simulink model "CB_sfun"  (R2024b)
settings: Solver=FixedStepDiscrete  StartTime=0.0  StopTime=inf  RelTol=1e-3  EnableMultiTasking=on
values from neighbouring files (symbols this model uses):
  cblc_battChargingMode = 5    [CB_ini.m]
  cblc_deltaSocThreshBalance = 0.1    [CB_ini.m]
  cblc_socThreshBalance = 50    [CB_ini.m]
settings Model: TunableVars=cblc_battChargingMode,cblc_deltaSocThreshBalance,cblc_socThreshBalance,cblc_voltThreshBalance  TunableVarsStorageClass=Auto,Auto,Auto,Auto  TunableVarsTypeQualifier=,,,  Creator=nctzv8  LastModifiedBy=voillat
settings ConfigSet: Description=OpenECU configuration set for code generation under RTW-EC.
settings SolverCC: AlgebraicLoopSolver=TrustRegion  PositivePriorityOrder=on
settings DataIOCC: LimitDataPoints=on  SaveFormat=Array  SignalLoggingSaveFormat=ModelDataLogs
settings OptimizationCC: DefaultParameterBehavior=Inlined  InlineInvariantSignals=on  ExpressionDepthLimit=2147483647  StateBitsets=on  DataBitsets=on  ZeroExternalMemoryAtStartup=off  ZeroInternalMemoryAtStartup=off  NoFixptDivByZeroProtection=on  EfficientFloat2IntCast=on  LifeSpan=1  EfficientTunableParamExpr=on
settings DebuggingCC: SaveWithParameterizedLinksMsg=none  SignalResolutionControl=TryResolveAllWithWarning  MultiTaskDSMMsg=warning  MultiTaskCondExecSysMsg=none  SingleTaskRateTransMsg=error  CheckMatrixSingularityMsg=warning  VectorMatrixConversionMsg=warning  SignalLabelMismatchMsg=warning  UnconnectedInputMsg=warning  UnconnectedOutputMsg=warning  UnconnectedLineMsg=warning  AllowSymbolicDim=off  StateNameClashWarn=warning  SFUnexpectedBacktrackingDiag=warning  SFNoUnconditionalDefaultTransitionDiag=warning  SFExecutionAtInitializationDiag=none  ArithmeticOperatorsInVariantConditions=warning
settings HardwareCC: ProdBitPerPointer=32  ProdBitPerSizeT=32  ProdBitPerPtrDiffT=32  ProdLargestAtomicInteger=Long  ProdLargestAtomicFloat=Double  ProdEndianess=BigEndian  ProdWordSize=32  ProdHWDeviceType=Freescale->32-bit PowerPC  TargetIntDivRoundTo=Zero  TargetEndianess=BigEndian  TargetHWDeviceType=Freescale->32-bit PowerPC  ProdEqTarget=off
settings ModelReferenceCC: EnableRefExpFcnMdlSchedulingChecks=on  PropagateSignalLabelsOutOfModel=off
settings SFSimCC: SimUseLocalCustomCode=off  MATLABDynamicMemAlloc=off  CustomCodeUndefinedFunction=UseInterfaceOnly
settings RTWCC: Description=OpenECU Platform Target (ERT, optimised floating-point code)  SystemTargetFile=openecu_ert.tlc  MakeCommand=make_rtw optimized_floating_point=1  TemplateMakefile=openecu_ert_r2015b_64.tmf  RetainRTWFile=on  RTWUseLocalCustomCode=off  IncludeHyperlinkInReport=on  GPUComputeCapability=3.5
settings CodeAppCC: ForceParamTrailComments=on  IgnoreCustomStorageClasses=off  SimulinkDataObjDesc=on  CustomSymbolStrType=$N$R$M  InsertBlockDesc=on  StateflowObjectComments=on  InternalIdentifier=Classic
settings STFCustomTargetCC: TargetLibSuffix=.a  GenerateSampleERTMain=on  IncludeMdlTerminateFcn=off  CombineOutputUpdateFcns=on  IncludeFileDelimiter=UseQuote  ERTCustomFileBanners=on  SupportContinuousTime=off  RemoveResetFunc=on  MATLABClassNameForMDSCustomization=Simulink.SoftwareTarget.ERTCustomization  SystemTargetFile=openecu_ert.tlc
settings ERTTargetCC: MultiwordLength=2048  GenerateSampleERTMain=on  ParMdlRefBuildCompliant=off  CompOptLevelCompliant=off  ConcurrentExecutionCompliant=off  IncludeMdlTerminateFcn=off  IncludeFileDelimiter=UseQuote  SupportNonInlinedSFcns=on  ModelStepFunctionPrototypeControlCompliant=off  CPPClassGenCompliant=off  UseToolchainInfoCompliant=off  ExtModeMexFile=noextcomm  ERTSrcFileBannerTemplate=oe_code_c_template.cgt  ERTHdrFileBannerTemplate=oe_code_h_template.cgt  ERTDataSrcFileTemplate=oe_data_c_template.cgt  ERTDataHdrFileTemplate=oe_data_h_template.cgt  ERTCustomFileTemplate=example_file_process.tlc  GlobalDataDefinition=InSeparateSourceFile  GlobalDataReference=InSeparateHeaderFile  ConvertIfToSwitch=off  SuppressUnreachableDefaultCases=off  EnableUserReplacementTypes=on  DynamicArrayContainerType=coder::array
settings ConfigComp: CovMetricSettings=dw  CovSaveCumulativeToWorkspaceVar=on  CovSaveSingleToWorkspaceVar=on  CovExternalEMLEnable=off

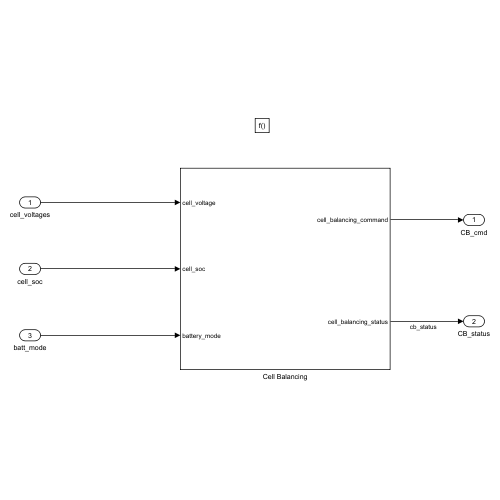
[thumbnail: Simulink's stored preview of the top-level diagram]
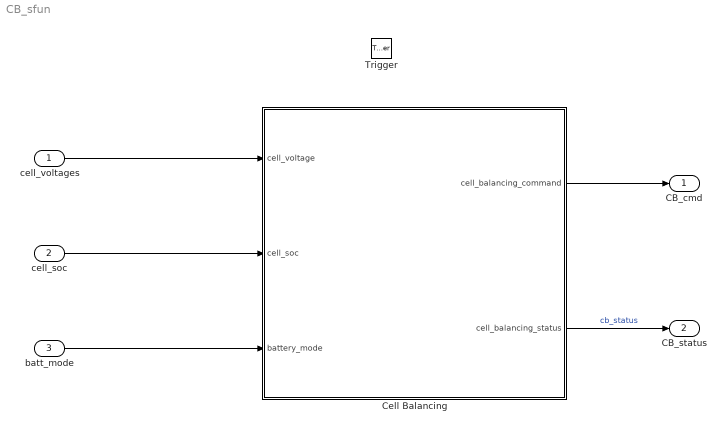
== system CB_sfun ==
  cell_voltages : Inport
  cell_soc : Inport  Port=2
  batt_mode : Inport  Port=3  OutDataTypeStr=uint8
  Trigger : TriggerPort  TriggerType=function-call  VariantControl=(inherit)  PortDimensions=1
  Cell Balancing : Subsystem  mask{sfcnParam1=cblc_battChargingMode, sfcnParam2=cblc_deltaSocThreshBalance, sfcnParam3=cblc_socThreshBalance}
      mask prompts: sfcnParam1 "cblc_battChargingMode:"; sfcnParam2 "cblc_deltaSocThreshBalance:"; sfcnParam3 "cblc_socThreshBalance:"
      mask help: Simulink:masks:GenSFuncDesc_MD
      mask Help: eval('feval(''rtwprivate'',''rtwhelpview'',''rtw_sfcn_block'')');
  CB_cmd : Outport
  CB_status : Outport  Port=2
  wires:
  cell_voltages/1 -> Cell Balancing/1(cell_voltage)
  batt_mode/1 -> Cell Balancing/3(battery_mode)
  cell_soc/1 -> Cell Balancing/2(cell_soc)
  Cell Balancing/1(cell_balancing_command) -> CB_cmd/1
  Cell Balancing/2(cell_balancing_status) -> CB_status/1  "cb_status"

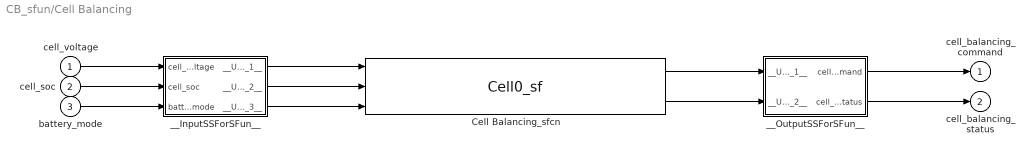
== system CB_sfun/Cell Balancing ==
  cell_voltage : Inport  PortDimensions=40
  cell_soc : Inport  Port=2  PortDimensions=40
  battery_mode : Inport  Port=3
  Cell Balancing_sfcn : S-Function  FunctionName=Cell0_sf  Parameters=sfcnParam1, sfcnParam2, sfcnParam3  SFunctionModules=""  SFunctionDeploymentMode=off  EnableBusSupport=off  mask{rtw_sf_name=Cell0_sf, showVar=off, sfcnParam1=sfcnParam1, sfcnParam2=sfcnParam2, sfcnParam3=sfcnParam3}
      mask prompts: rtw_sf_name "Simulink:masks:GenSFuncName_MP"; showVar "Simulink:masks:GenSFuncShowModuleList_MP"; sfcnParam1 "cblc_battChargingMode:"; sfcnParam2 "cblc_deltaSocThreshBalance:"; sfcnParam3 "cblc_socThreshBalance:"
      mask help: Simulink:masks:GenSFuncDesc_MD
      mask init:
      | displist = '';
      | if ~strcmp(get_param(gcb, 'FunctionName'), rtw_sf_name);
      |   set_param(gcb, 'FunctionName', rtw_sf_name);
      | end
      | % Check if we are generating code
      | rtw_mode = false;
      | if strcmpi(get_param(bdroot(gcb),'SimulationStatus'),'Initializing')
      | 	rtw_mode = strcmpi(get_param(bdroot(gcb),'BuildingRTWCode'),'on') && ...
      | 		~strcmpi(get_param(bdroot(gcb),'TargetStyle'),'SimulationTarget');
      | end
      | if showVar || rtw_mode
      | 	if exist('rtwsfunc') == 2 | exist('rtwsfunc') == 6
      | 		tmplist = rtwsfunc(rtw_sf_name,gcb);
      | 		tmplist = DAStudio.message('Simulink:masks:GenSFuncListOfModules_IC', tmplist);
      | 	elseif showVar
      | 		tmplist1 = DAStudio.message('Simulink:masks:GenSFuncListOfModules_IC', '');
      |         tmplist2 = DAStudio.message('Simulink:masks:GenSFuncNotLicensed_IC');
      |         tmplist = [tmplist1 tmplist2];
      |  	end
      | end
      | if showVar
      |   displist = tmplist;
      | end
      settings: CopyFcn=|
      | if ~strcmp(get_param(gcb,'Linkstatus'),'none') && ...
      | ~strcmp(get_param(gcb,'Linkstatus'),'implicit')
      |   set_param(gcb,'LinkStatus','none');
      | end
      mask Help: eval('feval(''rtwprivate'',''rtwhelpview'',''rtw_sfcn_block'')');
      mask Display:
      | port_label('input',1,'cell_voltage');
      | port_label('input',2,'cell_soc');
      | port_label('input',3,'battery_mode');
      | port_label('output',1,'cell_balancing_command');
      | port_label('output',2,'cell_balancing_status');
  __InputSSForSFun__ : Subsystem
  __OutputSSForSFun__ : Subsystem
  cell_balancing_command : Outport
  cell_balancing_status : Outport  Port=2
  wires:
  cell_voltage/1 -> __InputSSForSFun__/1(cell_voltage)
  cell_soc/1 -> __InputSSForSFun__/2(cell_soc)
  battery_mode/1 -> __InputSSForSFun__/3(battery_mode)
  __InputSSForSFun__/1(__UniqueOutportName__1__) -> Cell Balancing_sfcn/1
  __InputSSForSFun__/2(__UniqueOutportName__2__) -> Cell Balancing_sfcn/2
  __InputSSForSFun__/3(__UniqueOutportName__3__) -> Cell Balancing_sfcn/3
  Cell Balancing_sfcn/1 -> __OutputSSForSFun__/1(__UniqueInportName__1__)
  Cell Balancing_sfcn/2 -> __OutputSSForSFun__/2(__UniqueInportName__2__)
  __OutputSSForSFun__/1(cell_balancing_command) -> cell_balancing_command/1
  __OutputSSForSFun__/2(cell_balancing_status) -> cell_balancing_status/1

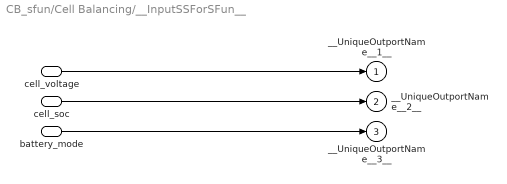
== system CB_sfun/Cell Balancing/__InputSSForSFun__ ==
  cell_voltage : Inport  PortDimensions=40
  cell_soc : Inport  Port=2  PortDimensions=40
  battery_mode : Inport  Port=3
  __UniqueOutportName__1__ : Outport
  __UniqueOutportName__2__ : Outport  Port=2
  __UniqueOutportName__3__ : Outport  Port=3
  wires:
  cell_voltage/1 -> __UniqueOutportName__1__/1
  cell_soc/1 -> __UniqueOutportName__2__/1
  battery_mode/1 -> __UniqueOutportName__3__/1

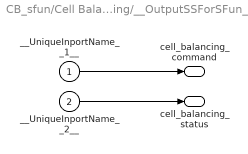
== system CB_sfun/Cell Balancing/__OutputSSForSFun__ ==
  __UniqueInportName__1__ : Inport
  __UniqueInportName__2__ : Inport  Port=2
  cell_balancing_command : Outport
  cell_balancing_status : Outport  Port=2
  wires:
  __UniqueInportName__1__/1 -> cell_balancing_command/1
  __UniqueInportName__2__/1 -> cell_balancing_status/1
